simulink model "Canard"  (R2023b)
settings: Solver=ode4  StartTime=0.0  StopTime=30  FixedStep=Step_Size  RelTol=1e-3
values from neighbouring files (symbols this model uses):
  I_TENSOR = [ I_xx,  0.0, -I_xz ... (first row only)    [aircraft_dynamics.m]    (also in duomian.m; main.m; parameters.m)
  Init_Euler = [0 5 0]*d2r    [duomian.m]    (also in main.m; parameters.m)
  Init_Pos = [0 0 0]    [duomian.m]    (also in main.m; parameters.m)
  Init_Rate = [0 0 0]*d2r    [duomian.m]    (also in main.m; parameters.m)
  Init_Vel = [18.6923 0 1.6352]    [duomian.m]    (also in main.m; parameters.m)
  Mass = 18    [aircraft_dynamics.m]    (also in duomian.m; main.m; parameters.m)
  max_T = 97.02    [duomian.m]    (also in main.m; parameters.m)
  min_T = 0    [duomian.m]    (also in main.m; parameters.m)
undefined symbols (not defined in the file or in its folder): deg, e0_0, e1_0, e2_0, e3_0, Earth, rad, s, WGS84
libraries: aerolibconvert2 x5, shared6dof x4, aerolibasang x4, sharedtransform x3, slpidlib x1, shared6dofsys x1, sharedutil x1, aerolibtransform2 x1, aerolibatmos2 x1
settings Model: PauseTimes=0.01  Creator=11851  LastModifiedBy=11851
settings DataIOCC: ExternalInput=getinputstruct(op_trim5)  InitialState=getstatestruct(op_trim5)

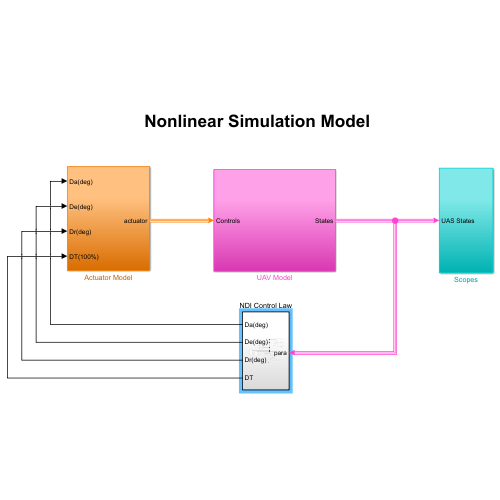
[thumbnail: Simulink's stored preview of the top-level diagram]
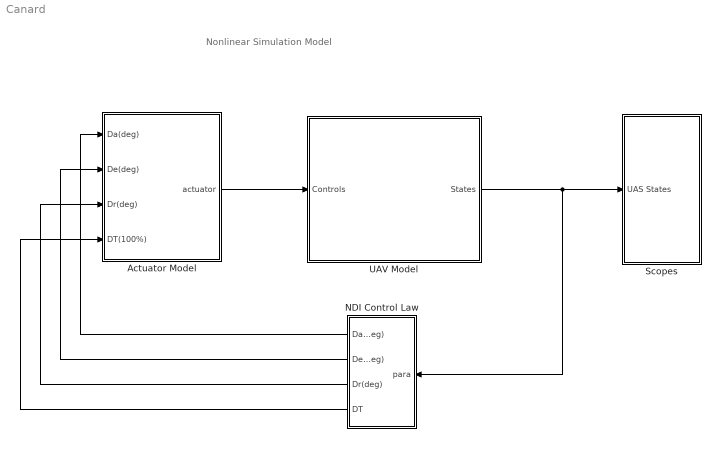
== system Canard ==
  note: Nonlinear Simulation Model
  Actuator Model : Subsystem
  NDI Control Law : Subsystem
  Scopes : Subsystem
  UAV Model : Subsystem
  wires:
  Actuator Model/1(actuator) -> UAV Model/1(Controls)
  UAV Model/1(States) -> NDI Control Law/1(para), Scopes/1(UAS States)
  NDI Control Law/1(Da(deg)) -> Actuator Model/1(Da(deg))
  NDI Control Law/2(De(deg)) -> Actuator Model/2(De(deg))
  NDI Control Law/3(Dr(deg)) -> Actuator Model/3(Dr(deg))
  NDI Control Law/4(DT) -> Actuator Model/4(DT(100%))

== system Canard/Actuator Model ==
  note: Actuator Models
  Da(deg) : Inport
  De(deg) : Inport  Port=2
  Dr(deg) : Inport  Port=3
  DT(100%) : Inport  Port=4
  Bus Creator : BusCreator  Inputs=2
  engine : Subsystem
  surface : Subsystem
  actuator : Outport
  wires:
  surface/1(control_surface(deg)) -> Bus Creator/1
  Bus Creator/1 -> actuator/1  "actuator"
  engine/1(throttle(100%)) -> Bus Creator/2
  Da(deg)/1 -> surface/1(Da(deg))
  De(deg)/1 -> surface/2(De(deg))
  DT(100%)/1 -> engine/1(DT(100%))
  Dr(deg)/1 -> surface/3(Dr(deg))

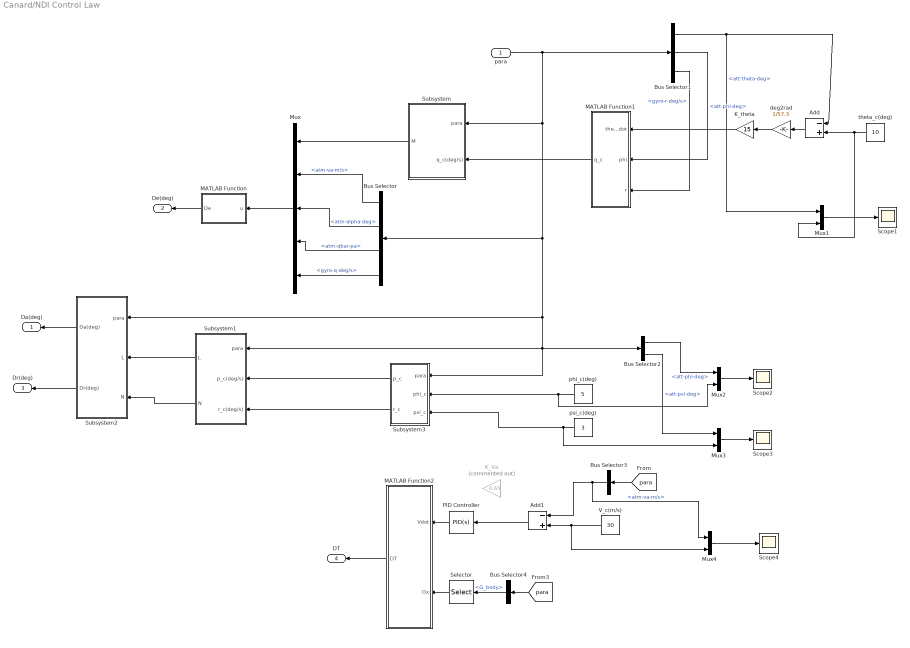
== system Canard/NDI Control Law ==
  para : Inport
  Add : Sum  Inputs=-+
  Add1 : Sum  Inputs=-+
  Bus Selector : BusSelector  OutputSignals=atm-va-m/s,atm-alpha-deg,atm-qbar-pa,gyro-q-deg/s
  Bus Selector1 : BusSelector  OutputSignals=att-theta-deg,att-phi-deg,gyro-r-deg/s
  Bus Selector2 : BusSelector  OutputSignals=att-phi-deg,att-psi-deg
  Bus Selector3 : BusSelector  OutputSignals=atm-va-m/s
  Bus Selector4 : BusSelector  OutputSignals=G_body
  K_Va : Gain  Commented=on  Gain=0.65
  K_theta : Gain  Gain=15
  MATLAB Function : MATLAB Function  TreatAsAtomicUnit=on
  MATLAB Function1 : MATLAB Function  TreatAsAtomicUnit=on
  MATLAB Function2 : MATLAB Function  TreatAsAtomicUnit=on
  Mux : Mux  Inputs=5
  Mux{1..4} (4 alike) : Mux  Inputs=2
  PID Controller : slpidlib/PID Controller  Controller=PID  Form=Parallel  TimeDomain=Continuous-time  UseExternalTs=off  SampleTime=-1  IntegratorMethod=Forward Euler  FilterMethod=Forward Euler  ControllerParametersSource=internal  P=0.75  I=0.05  UseKiTs=off  D=0  N=100  UseFilter=on  TunerSelectOption=Transfer Function Based (PID Tuner App)  InitialConditionSource=internal  InitialConditionForIntegrator=0  InitialConditionForFilter=0  DifferentiatorICPrevScaledInput=0  ExternalReset=none  TrackingMode=off  Kt=1  LimitOutput=off  SatLimitsSource=internal  UpperSaturationLimit=inf  LowerSaturationLimit=-inf  LinearizeAsGain=on  AntiWindupMode=none  Kb=1  LimitIntegrator=off  UpperIntegratorSaturationLimit=inf  LowerIntegratorSaturationLimit=-inf  POutMin=[]  POutMax=[]  IOutMin=[]  IOutMax=[]  DOutMin=[]  DOutMax=[]  NOutMin=[]  NOutMax=[]  SumOutMin=[]  SumOutMax=[]  SaturationOutMin=[]  SaturationOutMax=[]  PParamMin=[]  PParamMax=[]  IParamMin=[]  IParamMax=[]  DParamMin=[]  DParamMax=[]  NParamMin=[]  NParamMax=[]  KbParamMin=[]  KbParamMax=[]  KtParamMin=[]  KtParamMax=[]  KbOutMin=[]  KbOutMax=[]  KtOutMin=[]  KtOutMax=[]  IntegratorOutMin=[]  IntegratorOutMax=[]  FilterOutMin=[]  FilterOutMax=[]  SumI1OutMin=[]  SumI1OutMax=[]  SumI2OutMin=[]  SumI2OutMax=[]  SumI3OutMin=[]  SumI3OutMax=[]  SumI4OutMin=[]  SumI4OutMax=[]  SumDOutMin=[]  SumDOutMax=[]  DifferentiatorOutMin=[]  DifferentiatorOutMax=[]  FilterDiffOutCoefMin=[]  FilterDiffOutCoefMax=[]  ReciprocalOutMin=[]  ReciprocalOutMax=[]  SumDenOutMin=[]  SumDenOutMax=[]  SumNumOutMin=[]  SumNumOutMax=[]  DivideOutMin=[]  DivideOutMax=[]  UdiffTsProdOutMin=[]  UdiffTsProdOutMax=[]  NTsProdOutMin=[]  NTsProdOutMax=[]  UintegralTsProdOutMin=[]  UintegralTsProdOutMax=[]  UngainTsProdOutMin=[]  UngainTsProdOutMax=[]  ClampingZeroOutDataTypeStr=Inherit: Inherit via back propagation  ClampingZeroOutMin=[]  ClampingZeroOutMax=[]  FilterDenConstantOutDataTypeStr=Inherit: Inherit via back propagation  FilterDenConstantOutMin=[]  FilterDenConstantOutMax=[]  PCopyOutDataTypeStr=Inherit: Inherit via back propagation  PCopyOutMin=[]  PCopyOutMax=[]  NCopyOutDataTypeStr=Inherit: Inherit via back propagation  NCopyOutMin=[]  NCopyOutMax=[]  IntegratorContinuousStateAttributes=''  IntegratorStateMustResolveToSignalObject=off  IntegratorRTWStateStorageClass=Auto  FilterContinuousStateAttributes=''  FilterStateMustResolveToSignalObject=off  FilterRTWStateStorageClass=Auto  ParallelPVariant=InternalParameters  IdealPVariant=Disabled  IVariant=InternalParameters  DVariant=InternalParameters  IntegratorVariant=Continuous  SatVariant=Disabled  AWVariant=Passthrough  PCopyVariant=Disabled  TRVariant=Disabled  FdbkBlocksVariant=Forward  IdealPFdbkVariant=Disabled  SatFdbkVariant=Disabled  DerivativeFilterVariant=ContFilter  NVariant=InternalParameters  NCopyVariant=Disabled  FilterICVariant=InternalICsFilter  IntegratorICVariant=InternalICs  ExternalResetVariant=Disabled  TRSumVariant=Passthrough  SumFdbkVariant=Disabled  SumVariant=Sum_PID  TsampFilterVariant=InternalTs  TsampNgainVariant=Passthrough  TsampIntegralVariant=Disabled_SignalSpec  ExternalSaturationOutDataTypeStr=Inherit: Same as second input
  Scope{1..4} (4 alike) : Scope
  Selector : Selector  InputPortWidth=3  IndexOptions=Index vector (dialog)  Indices=1  OutputSizes=1
  Subsystem : Subsystem
  Subsystem1 : Subsystem
  Subsystem2 : Subsystem
  Subsystem3 : Subsystem
  V_c(m/s) : Constant  Value=30
  deg2rad : Gain  Gain=1/57.3
  phi_c(deg) : Constant  Value=5
  psi_c(deg) : Constant  Value=3
  theta_c(deg) : Constant  Value=10
  Da(deg) : Outport
  De(deg) : Outport  Port=2
  Dr(deg) : Outport  Port=3
  DT : Outport  Port=4
  wires:
  Subsystem1/2(N) -> Subsystem2/3(N)
  Mux4/1 -> Scope4/1
  Bus Selector2/1 -> Mux2/1  "<att-phi-deg>"
  Bus Selector1/1 -> Mux1/1, Add/1  "<att-theta-deg>"
  deg2rad/1 -> K_theta/1
  [para] -> Bus Selector3/1
  Bus Selector3/1 -> Mux4/1, Add1/1  "<atm-va-m/s>"
  para/1 -> Subsystem3/1(para), Bus Selector2/1, Subsystem1/1(para), Subsystem2/1(para), Bus Selector/1, Subsystem/1(para), Bus Selector1/1
  Bus Selector2/2 -> Mux3/1  "<att-psi-deg>"
  Subsystem1/1(L) -> Subsystem2/2(L)
  Add/1 -> deg2rad/1
  Subsystem/1(M) -> Mux/1
  theta_c(deg)/1 -> Mux1/2, Add/2
  Bus Selector1/3 -> MATLAB Function1/3(r)  "<gyro-r-deg/s>"
  Subsystem3/2(r_c) -> Subsystem1/3(r_c(deg/s))
  Mux2/1 -> Scope2/1
  Mux1/1 -> Scope1/1
  K_theta/1 -> MATLAB Function1/1(thetac_dot)
  MATLAB Function1/1(q_c) -> Subsystem/2(q_c(deg/s))
  [para] -> Bus Selector4/1
  psi_c(deg)/1 -> Mux3/2, Subsystem3/3(psi_c)
  Bus Selector/4 -> Mux/5  "<gyro-q-deg/s>"
  Mux/1 -> MATLAB Function/1(u)
  Subsystem3/1(p_c) -> Subsystem1/2(p_c(deg/s))
  Bus Selector/2 -> Mux/3  "<atm-alpha-deg>"
  Mux3/1 -> Scope3/1
  phi_c(deg)/1 -> Mux2/2, Subsystem3/2(phi_c)
  Bus Selector4/1 -> Selector/1  "<G_body>"
  Bus Selector/3 -> Mux/4  "<atm-qbar-pa>"
  Bus Selector1/2 -> MATLAB Function1/2(phi)  "<att-phi-deg>"
  Bus Selector/1 -> Mux/2  "<atm-va-m/s>"
  V_c(m/s)/1 -> Mux4/2, Add1/2
  Selector/1 -> MATLAB Function2/2(Gx)
  MATLAB Function2/1(DT) -> DT/1
  Subsystem2/2(Dr(deg)) -> Dr(deg)/1
  MATLAB Function/1(De) -> De(deg)/1
  Subsystem2/1(Da(deg)) -> Da(deg)/1
  Add1/1 -> PID Controller/1
  PID Controller/1 -> MATLAB Function2/1(Vdot)

== system Canard/Scopes ==
  UAS States : Inport
  Bus Selector : BusSelector  OutputSignals=att-phi-deg,att-theta-deg,att-psi-deg,gyro-p-deg/s,gyro-q-deg/s,gyro-r-deg/s,atm-va-m/s,atm-alpha-deg,atm-beta-deg
  Euler : Scope  NumInputPorts=3
  Vabs : Scope
  alpha_beta : Scope  NumInputPorts=2
  pqr : Scope  NumInputPorts=3
  wires:
  UAS States/1 -> Bus Selector/1
  Bus Selector/1 -> Euler/1  "<att-phi-deg>"
  Bus Selector/2 -> Euler/2  "<att-theta-deg>"
  Bus Selector/3 -> Euler/3  "<att-psi-deg>"
  Bus Selector/4 -> pqr/1  "<gyro-p-deg/s>"
  Bus Selector/5 -> pqr/2  "<gyro-q-deg/s>"
  Bus Selector/6 -> pqr/3  "<gyro-r-deg/s>"
  Bus Selector/7 -> Vabs/1  "<atm-va-m/s>"
  Bus Selector/8 -> alpha_beta/1  "<atm-alpha-deg>"
  Bus Selector/9 -> alpha_beta/2  "<atm-beta-deg>"

== system Canard/UAV Model ==
  note: Dynamics Model
  Controls : Inport
  Aerodynamics : Subsystem
  Bus Creator : BusCreator  Inputs=2
  Equations of Motion : Subsystem
  Propulsive Force & Moment : Subsystem
  Total Force & Moment : Subsystem
  environment : Subsystem
  gravitation : Subsystem
  States : Outport
  tag scope: para=global
  wires:
  Aerodynamics/1(fxyz) -> Total Force & Moment/1(F_aero)
  Aerodynamics/2(mxyz) -> Total Force & Moment/2(M_aero)
  Controls/1 -> Propulsive Force & Moment/1(Controls), Bus Creator/1
  Propulsive Force & Moment/1(F_prop) -> Total Force & Moment/3(F_prop)
  Propulsive Force & Moment/2(M_prop) -> Total Force & Moment/4(M_prop)
  Total Force & Moment/1(F_cg) -> Equations of Motion/1(Force)
  Total Force & Moment/2(M_cg) -> Equations of Motion/2(Moment)
  Equations of Motion/1(para) -> States/1, Bus Creator/2, gravitation/1(state), [para]
  gravitation/1(gravity) -> Total Force & Moment/5(gravity)
  gravitation/2(moment) -> Total Force & Moment/6(M_grav)
  Bus Creator/1 -> Aerodynamics/1(state)

== system Canard/Actuator Model/engine ==
  note: 发动机油门开合度
  DT(100%) : Inport
  Gain : Gain  Gain=10
  Integrator : Integrator  InitialConditionSource=external
  Saturation1 : Saturate  UpperLimit=300  LowerLimit=-300
  Saturation2 : Saturate  UpperLimit=1  LowerLimit=0
  Sum : Sum  Inputs=|+-
  throttle(100%) : Outport
  wires:
  Integrator/1 -> Saturation2/1
  Saturation1/1 -> Integrator/1
  Gain/1 -> Saturation1/1
  Sum/1 -> Gain/1
  DT(100%)/1 -> Sum/1, Integrator/2
  Saturation2/1 -> throttle(100%)/1, Sum/2  "throttle"

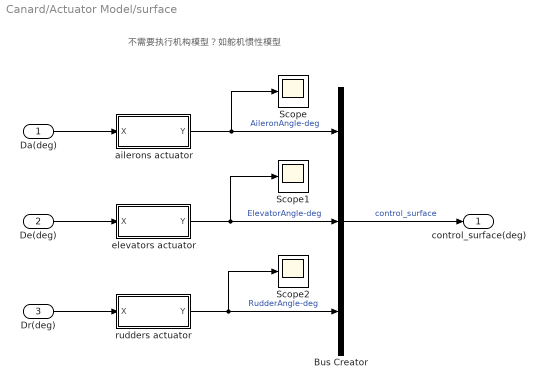
== system Canard/Actuator Model/surface ==
  note: 不需要执行机构模型？如舵机惯性模型
  Da(deg) : Inport
  De(deg) : Inport  Port=2
  Dr(deg) : Inport  Port=3
  Bus Creator : BusCreator  Inputs=3
  Scope : Scope
  Scope1 : Scope
  Scope2 : Scope
  ailerons actuator : Subsystem
  elevators actuator : Subsystem
  rudders actuator : Subsystem
  control_surface(deg) : Outport
  wires:
  Bus Creator/1 -> control_surface(deg)/1  "control_surface"
  ailerons actuator/1(Y) -> Scope/1, Bus Creator/1  "AileronAngle-deg"
  elevators actuator/1(Y) -> Scope1/1, Bus Creator/2  "ElevatorAngle-deg"
  rudders actuator/1(Y) -> Scope2/1, Bus Creator/3  "RudderAngle-deg"
  Da(deg)/1 -> ailerons actuator/1(X)
  De(deg)/1 -> elevators actuator/1(X)
  Dr(deg)/1 -> rudders actuator/1(X)

== system Canard/NDI Control Law/Subsystem ==
  para : Inport
  q_c(deg/s) : Inport  Port=2
  Add : Sum  Inputs=-+
  Bus Selector : BusSelector  OutputSignals=gyro-p-deg/s,gyro-q-deg/s,gyro-r-deg/s
  K_q : Gain  Gain=5
  MATLAB Function : MATLAB Function  TreatAsAtomicUnit=on
  deg2rad : Gain  Gain=1/57.3
  deg2rad1 : Gain  Gain=1/57.3
  deg2rad2 : Gain  Gain=1/57.3
  M : Outport
  wires:
  para/1 -> Bus Selector/1
  Bus Selector/2 -> Add/1  "<gyro-q-deg/s>"
  q_c(deg/s)/1 -> Add/2
  deg2rad/1 -> K_q/1
  Add/1 -> deg2rad/1
  K_q/1 -> MATLAB Function/3(q_dot)
  Bus Selector/1 -> deg2rad2/1  "<gyro-p-deg/s>"
  Bus Selector/3 -> deg2rad1/1  "<gyro-r-deg/s>"
  MATLAB Function/1(M) -> M/1
  deg2rad2/1 -> MATLAB Function/1(p)
  deg2rad1/1 -> MATLAB Function/2(r)

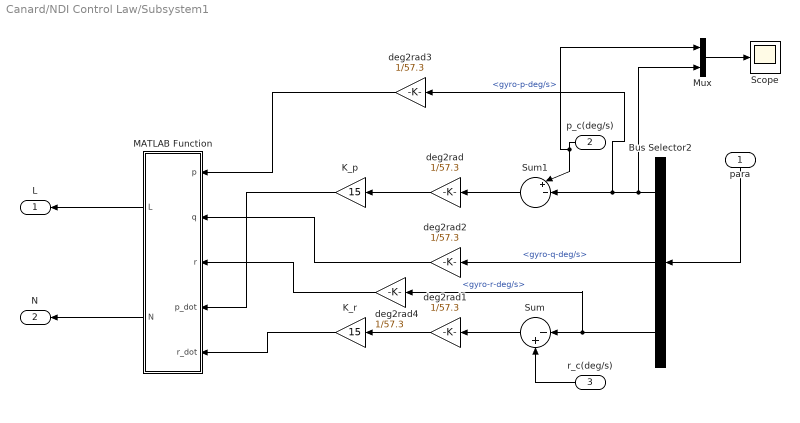
== system Canard/NDI Control Law/Subsystem1 ==
  para : Inport
  p_c(deg/s) : Inport  Port=2
  r_c(deg/s) : Inport  Port=3
  Bus Selector2 : BusSelector  OutputSignals=gyro-p-deg/s,gyro-q-deg/s,gyro-r-deg/s
  K_p : Gain  Gain=15
  K_r : Gain  Gain=15
  MATLAB Function : MATLAB Function  TreatAsAtomicUnit=on
  Mux : Mux  Inputs=2
  Scope : Scope
  Sum : Sum  Inputs=|-+
  Sum1 : Sum  Inputs=|+-||
  deg2rad{,1..4} (5 alike) : Gain  Gain=1/57.3
  L : Outport
  N : Outport  Port=2
  wires:
  Bus Selector2/2 -> deg2rad2/1  "<gyro-q-deg/s>"
  r_c(deg/s)/1 -> Sum/2
  para/1 -> Bus Selector2/1
  deg2rad1/1 -> K_r/1
  deg2rad/1 -> K_p/1
  Bus Selector2/1 -> Mux/2, deg2rad3/1, Sum1/2  "<gyro-p-deg/s>"
  Bus Selector2/3 -> deg2rad4/1, Sum/1  "<gyro-r-deg/s>"
  Sum1/1 -> deg2rad/1
  Sum/1 -> deg2rad1/1
  p_c(deg/s)/1 -> Sum1/1, Mux/1
  deg2rad3/1 -> MATLAB Function/1(p)
  deg2rad2/1 -> MATLAB Function/2(q)
  deg2rad4/1 -> MATLAB Function/3(r)
  K_p/1 -> MATLAB Function/4(p_dot)
  K_r/1 -> MATLAB Function/5(r_dot)
  MATLAB Function/1(L) -> L/1
  MATLAB Function/2(N) -> N/1
  Mux/1 -> Scope/1

== system Canard/NDI Control Law/Subsystem2 ==
  para : Inport
  L : Inport  Port=2
  N : Inport  Port=3
  Bus Selector2 : BusSelector  OutputSignals=atm-qbar-pa,atm-alpha-deg,atm-beta-deg,atm-va-m/s,gyro-p-deg/s,gyro-r-deg/s
  MATLAB Function : MATLAB Function  TreatAsAtomicUnit=on
  Da(deg) : Outport
  Dr(deg) : Outport  Port=2
  wires:
  para/1 -> Bus Selector2/1
  Bus Selector2/1 -> MATLAB Function/1(qbar)  "<atm-qbar-pa>"
  Bus Selector2/2 -> MATLAB Function/2(alpha)  "<atm-alpha-deg>"
  Bus Selector2/4 -> MATLAB Function/4(va)  "<atm-va-m/s>"
  Bus Selector2/3 -> MATLAB Function/3(beta)  "<atm-beta-deg>"
  Bus Selector2/6 -> MATLAB Function/6(r)  "<gyro-r-deg/s>"
  Bus Selector2/5 -> MATLAB Function/5(p)  "<gyro-p-deg/s>"
  L/1 -> MATLAB Function/7(L)
  N/1 -> MATLAB Function/8(N)
  MATLAB Function/2(Dr) -> Dr(deg)/1
  MATLAB Function/1(Da) -> Da(deg)/1

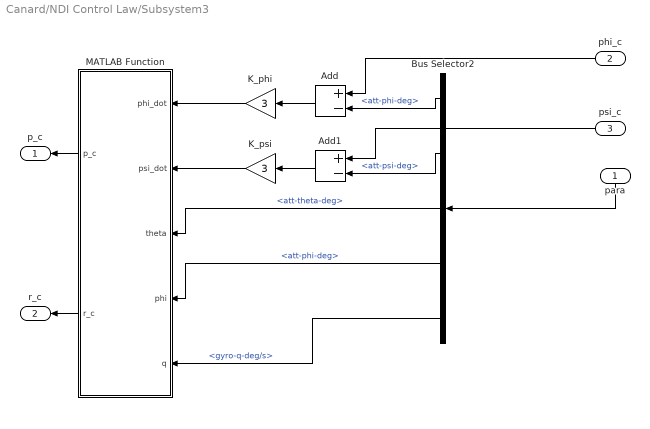
== system Canard/NDI Control Law/Subsystem3 ==
  para : Inport
  phi_c : Inport  Port=2
  psi_c : Inport  Port=3
  Add : Sum  Inputs=+-
  Add1 : Sum  Inputs=+-
  Bus Selector2 : BusSelector  OutputSignals=att-phi-deg,att-psi-deg,att-theta-deg,att-phi-deg,gyro-q-deg/s
  K_phi : Gain  Gain=3
  K_psi : Gain  Gain=3
  MATLAB Function : MATLAB Function  TreatAsAtomicUnit=on
  p_c : Outport
  r_c : Outport  Port=2
  wires:
  Bus Selector2/5 -> MATLAB Function/5(q)  "<gyro-q-deg/s>"
  para/1 -> Bus Selector2/1
  Bus Selector2/1 -> Add/2  "<att-phi-deg>"
  Bus Selector2/2 -> Add1/2  "<att-psi-deg>"
  Bus Selector2/3 -> MATLAB Function/3(theta)  "<att-theta-deg>"
  phi_c/1 -> Add/1
  Add/1 -> K_phi/1
  psi_c/1 -> Add1/1
  Add1/1 -> K_psi/1
  Bus Selector2/4 -> MATLAB Function/4(phi)  "<att-phi-deg>"
  MATLAB Function/1(p_c) -> p_c/1
  MATLAB Function/2(r_c) -> r_c/1
  K_phi/1 -> MATLAB Function/1(phi_dot)
  K_psi/1 -> MATLAB Function/2(psi_dot)

== system Canard/UAV Model/Aerodynamics ==
  note: Aerodynamics Module
  state : Inport
  Bus Selector : BusSelector  OutputSignals=actuator.control_surface.AileronAngle-deg,actuator.control_surface.ElevatorAngle-deg,actuator.control_surface.RudderAngle-deg,para.atm-alpha-deg,para.atm-beta-deg,para.gyro-p-deg/s,para.gyro-q-deg/s,para.gyro-r-deg/s,para.atm-va-m/s,para.atm-qbar-pa
  Demux : Demux  Outputs=6
  Mux : Mux  Inputs=10
  Mux1 : Mux  Inputs=3
  Mux2 : Mux  Inputs=3
  S-Function : S-Function  FunctionName=Canard_aero  SFunctionDeploymentMode=off  EnableBusSupport=off
  fxyz : Outport
  mxyz : Outport  Port=2
  wires:
  Bus Selector/9 -> Mux/9  "<atm-va-m/s>"
  Bus Selector/10 -> Mux/10  "<atm-qbar-pa>"
  Bus Selector/1 -> Mux/1  "<AileronAngle-deg>"
  Demux/2 -> Mux1/2
  Mux2/1 -> mxyz/1
  Demux/3 -> Mux1/3
  Demux/6 -> Mux2/3
  Bus Selector/5 -> Mux/5  "<atm-beta-deg>"
  Mux1/1 -> fxyz/1
  Demux/4 -> Mux2/1
  Mux/1 -> S-Function/1
  S-Function/1 -> Demux/1
  state/1 -> Bus Selector/1
  Bus Selector/2 -> Mux/2  "<ElevatorAngle-deg>"
  Demux/5 -> Mux2/2
  Bus Selector/7 -> Mux/7  "<gyro-q-deg/s>"
  Bus Selector/4 -> Mux/4  "<atm-alpha-deg>"
  Demux/1 -> Mux1/1
  Bus Selector/6 -> Mux/6  "<gyro-p-deg/s>"
  Bus Selector/3 -> Mux/3  "<RudderAngle-deg>"
  Bus Selector/8 -> Mux/8  "<gyro-r-deg/s>"

== system Canard/UAV Model/Equations of Motion ==
  note: 6DOF Motion of Equations
  Force : Inport  PortDimensions=3
  Moment : Inport  Port=2  PortDimensions=3
  Subsystem : Subsystem
  parameter : Subsystem
  para : Outport
  wires:
  Moment/1 -> Subsystem/2(Moments)
  Force/1 -> Subsystem/1(Forces)
  Subsystem/1(Ve) -> parameter/1(Ve)
  Subsystem/2(Xe) -> parameter/2(Xe)
  Subsystem/3(Euler) -> parameter/3(Euler)
  Subsystem/4(DCM) -> parameter/4(Rbe)
  Subsystem/5(Vb) -> parameter/5(Vb)
  Subsystem/6(p,q,r) -> parameter/6(ω)
  Subsystem/7(pdot,qdot,rdot) -> parameter/7(dω)
  Subsystem/8(Ab) -> parameter/8(Ab)
  parameter/1(para) -> para/1

== system Canard/UAV Model/Propulsive Force & Moment ==
  note: Propulsive Force and Moment
  Controls : Inport
  Bus Selector : BusSelector  OutputSignals=throttle
  Constant : Constant  Value=0
  Mux : Mux  Inputs=3
  Mux1 : Mux  Inputs=3
  Saturation : Saturate  UpperLimit=max_T  LowerLimit=min_T
  max_T : Gain  Gain=max_T
  F_prop : Outport
  M_prop : Outport  Port=2
  wires:
  Mux1/1 -> M_prop/1
  Constant/1 -> Mux1/3, Mux1/2, Mux1/1, Mux/3, Mux/2
  Controls/1 -> Bus Selector/1
  Mux/1 -> F_prop/1
  Saturation/1 -> Mux/1
  max_T/1 -> Saturation/1
  Bus Selector/1 -> max_T/1  "<throttle>"

== system Canard/UAV Model/Total Force & Moment ==
  note: Total Force and Moment
  F_aero : Inport  PortDimensions=3
  M_aero : Inport  Port=2  PortDimensions=3
  F_prop : Inport  Port=3  PortDimensions=3
  M_prop : Inport  Port=4  PortDimensions=3
  gravity : Inport  Port=5  PortDimensions=3
  M_grav : Inport  Port=6  PortDimensions=3
  Total Force : Sum  Inputs=+++  InputSameDT=on  SaturateOnIntegerOverflow=on  OutDataTypeStr=Inherit: Same as first input
  Total Moment : Sum  Inputs=+++  InputSameDT=on  SaturateOnIntegerOverflow=on  OutDataTypeStr=Inherit: Same as first input
  F_cg : Outport
  M_cg : Outport  Port=2
  wires:
  Total Force/1 -> F_cg/1
  F_aero/1 -> Total Force/1
  F_prop/1 -> Total Force/2
  M_prop/1 -> Total Moment/2
  Total Moment/1 -> M_cg/1
  M_aero/1 -> Total Moment/1
  gravity/1 -> Total Force/3
  M_grav/1 -> Total Moment/3

== system Canard/UAV Model/environment ==
  note: 物理环境模块，用于模拟飞机所处的环境，包括
      |
      | （1）标准大气模型
      | （2）风场运动模型，比如风切变等
      | （3）重力场模型
      | （4）磁力场模型
  Bus Creator1 : BusCreator  Inputs=4
  atmosphere : Subsystem
  gravity : Subsystem
  magnetic : Subsystem
  windshear : Subsystem
  tag scope: environment=global
  wires:
  Bus Creator1/1 -> [environment]  "Environment"
  atmosphere/1(atmo) -> Bus Creator1/1  "atmo"
  windshear/1(wind) -> Bus Creator1/2  "wind"
  gravity/1(g) -> Bus Creator1/3  "g"
  magnetic/1(mag) -> Bus Creator1/4  "mag"

== system Canard/UAV Model/gravitation ==
  state : Inport
  Bus Selector : BusSelector  OutputSignals=att-theta-deg,att-phi-deg
  Constant : Constant  Value=Mass
  Constant1 : Constant  Value=9.81
  MATLAB Function : MATLAB Function  TreatAsAtomicUnit=on
  Mux : Mux  Inputs=3
  Mux1 : Mux  Inputs=3
  Product : Product
  zero1 : Constant  Value=[0 0 0]
  gravity : Outport
  moment : Outport  Port=2
  wires:
  zero1/1 -> moment/1
  state/1 -> Bus Selector/1
  Bus Selector/1 -> Mux/2  "<att-theta-deg>"
  Bus Selector/2 -> Mux/3  "<att-phi-deg>"
  Constant/1 -> Product/1
  Product/1 -> Mux/1
  Mux/1 -> MATLAB Function/1(u)
  MATLAB Function/1(Gx) -> Mux1/1
  MATLAB Function/2(Gy) -> Mux1/2
  MATLAB Function/3(Gz) -> Mux1/3
  Mux1/1 -> gravity/1
  Constant1/1 -> Product/2

== system Canard/Actuator Model/surface/ailerons actuator ==
  X : Inport
  Gain : Gain  Gain=100
  Integrator : Integrator  InitialConditionSource=external
  Saturation1 : Saturate  UpperLimit=300  LowerLimit=-300
  Saturation2 : Saturate  UpperLimit=20  LowerLimit=-20
  Sum : Sum  Inputs=|+-
  Y : Outport
  wires:
  Integrator/1 -> Saturation2/1
  Saturation1/1 -> Integrator/1
  Gain/1 -> Saturation1/1
  Sum/1 -> Gain/1
  Saturation2/1 -> Y/1, Sum/2
  X/1 -> Sum/1, Integrator/2

== system Canard/Actuator Model/surface/elevators actuator ==
  X : Inport
  Gain : Gain  Gain=100
  Integrator : Integrator  InitialConditionSource=external  InitialCondition=0.811
  Saturation1 : Saturate  UpperLimit=300  LowerLimit=-300
  Saturation2 : Saturate  UpperLimit=20  LowerLimit=-20
  Scope : Scope
  Sum : Sum  Inputs=|+-
  Y : Outport
  wires:
  Integrator/1 -> Saturation2/1
  Saturation1/1 -> Integrator/1
  Gain/1 -> Saturation1/1
  Sum/1 -> Gain/1
  Saturation2/1 -> Scope/1, Y/1, Sum/2
  X/1 -> Integrator/2, Sum/1

== system Canard/Actuator Model/surface/rudders actuator ==
  X : Inport
  Gain : Gain  Gain=100
  Integrator : Integrator  InitialConditionSource=external
  Saturation1 : Saturate  UpperLimit=300  LowerLimit=-300
  Saturation2 : Saturate  UpperLimit=20  LowerLimit=-20
  Sum : Sum  Inputs=|+-
  Y : Outport
  wires:
  Integrator/1 -> Saturation2/1
  Saturation1/1 -> Integrator/1
  Gain/1 -> Saturation1/1
  Sum/1 -> Gain/1
  Saturation2/1 -> Y/1, Sum/2
  X/1 -> Sum/1, Integrator/2

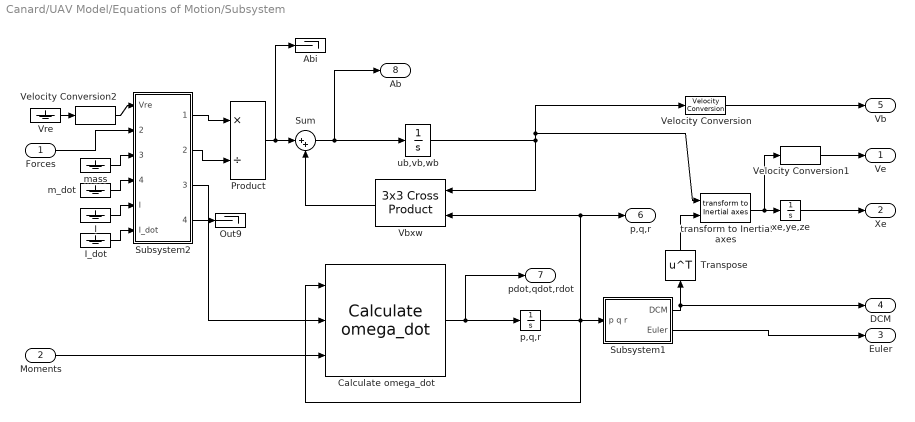
== system Canard/UAV Model/Equations of Motion/Subsystem ==
  Forces : Inport  OutDataTypeStr=double  Unit=N  PortDimensions=3
  Moments : Inport  Port=2  OutDataTypeStr=double  Unit=N*m  PortDimensions=3
  Abi : Terminator
  Calculate omega_dot : shared6dofsys/Calculate omega_dot  aMode=aMode
  I : Ground
  I_dot : Ground
  Out9 : Terminator
  Product : Product  Inputs=*/  SaturateOnIntegerOverflow=on  OutDataTypeStr=Inherit: Same as first input
  Subsystem1 : Subsystem
  Subsystem2 : Subsystem
  Sum : Sum  Inputs=|++  SaturateOnIntegerOverflow=on
  Transpose : Math  Operator=transpose  SignedPower=on
  Vbxw : sharedutil/3x3 Cross Product  aMode=aMode
  Velocity Conversion : shared6dof/6DOF (Euler Angles)/Velocity Conversion  SystemSampleTime=-1  VariantActivationTime=update diagram  AllowFlexibleInterface=on  Latency=0  AutoFrameSizeCalculation=off
  Velocity Conversion1 : shared6dof/6DOF (Euler Angles)/Velocity Conversion1  SystemSampleTime=-1  VariantActivationTime=update diagram  AllowFlexibleInterface=on  Latency=0  AutoFrameSizeCalculation=off
  Velocity Conversion2 : shared6dof/6DOF (Euler Angles)/Velocity Conversion2  SystemSampleTime=-1  VariantActivationTime=update diagram  AllowFlexibleInterface=on  Latency=0  AutoFrameSizeCalculation=off
  Vre : Ground
  m_dot : Ground
  mass : Ground
  "p,q,r " : Integrator  InitialCondition=Init_Rate
  "transform to Inertial axes " : shared6dof/6DOF (Euler Angles)/transform to Inertial axes   SystemSampleTime=-1  VariantActivationTime=update diagram  AllowFlexibleInterface=on  Latency=0  AutoFrameSizeCalculation=off
  ub,vb,wb : Integrator  InitialCondition=Init_Vel
  xe,ye,ze : Integrator  InitialCondition=Init_Pos
  Ve : Outport  OutDataTypeStr=double  Unit=m/s  VectorParamsAs1DForOutWhenUnconnected=off
  Xe : Outport  Port=2  OutDataTypeStr=double  Unit=m  VectorParamsAs1DForOutWhenUnconnected=off
  Euler : Outport  Port=3  OutDataTypeStr=double  Unit=rad  VectorParamsAs1DForOutWhenUnconnected=off
  DCM : Outport  Port=4  OutDataTypeStr=double  Unit=1  VectorParamsAs1DForOutWhenUnconnected=off
  Vb : Outport  Port=5  OutDataTypeStr=double  Unit=m/s  VectorParamsAs1DForOutWhenUnconnected=off
  p,q,r : Outport  Port=6  OutDataTypeStr=double  Unit=rad/s  VectorParamsAs1DForOutWhenUnconnected=off
  pdot,qdot,rdot : Outport  Port=7  OutDataTypeStr=double  Unit=rad/s^2  VectorParamsAs1DForOutWhenUnconnected=off
  Ab : Outport  Port=8  OutDataTypeStr=double  Unit=m/s^2  VectorParamsAs1DForOutWhenUnconnected=off
  wires:
  Transpose/1 -> "transform to Inertial axes "/2
  ub,vb,wb/1 -> Vbxw/1, Velocity Conversion/1, "transform to Inertial axes "/1
  m_dot/1 -> Subsystem2/4(m_dot)
  Calculate omega_dot/1 -> pdot,qdot,rdot/1, "p,q,r "/1
  I_dot/1 -> Subsystem2/6(I_dot)
  Forces/1 -> Subsystem2/2(forces)
  Product/1 -> Sum/1, Abi/1
  "p,q,r "/1 -> Calculate omega_dot/1, Subsystem1/1(p q r), p,q,r/1, Vbxw/2
  Vbxw/1 -> Sum/2
  Subsystem2/1("forces ") -> Product/1
  Sum/1 -> Ab/1, ub,vb,wb/1
  Moments/1 -> Calculate omega_dot/3
  Velocity Conversion/1 -> Vb/1
  Subsystem1/1(DCM) -> DCM/1, Transpose/1
  Subsystem1/2(Euler) -> Euler/1
  Velocity Conversion1/1 -> Ve/1
  mass/1 -> Subsystem2/3("mass ")
  Velocity Conversion2/1 -> Subsystem2/1(Vre)
  Vre/1 -> Velocity Conversion2/1
  "transform to Inertial axes "/1 -> xe,ye,ze/1, Velocity Conversion1/1
  xe,ye,ze/1 -> Xe/1
  I/1 -> Subsystem2/5(I)
  Subsystem2/4(Out9) -> Out9/1
  Subsystem2/3("inertia, 0") -> Calculate omega_dot/2
  Subsystem2/2(mass) -> Product/2

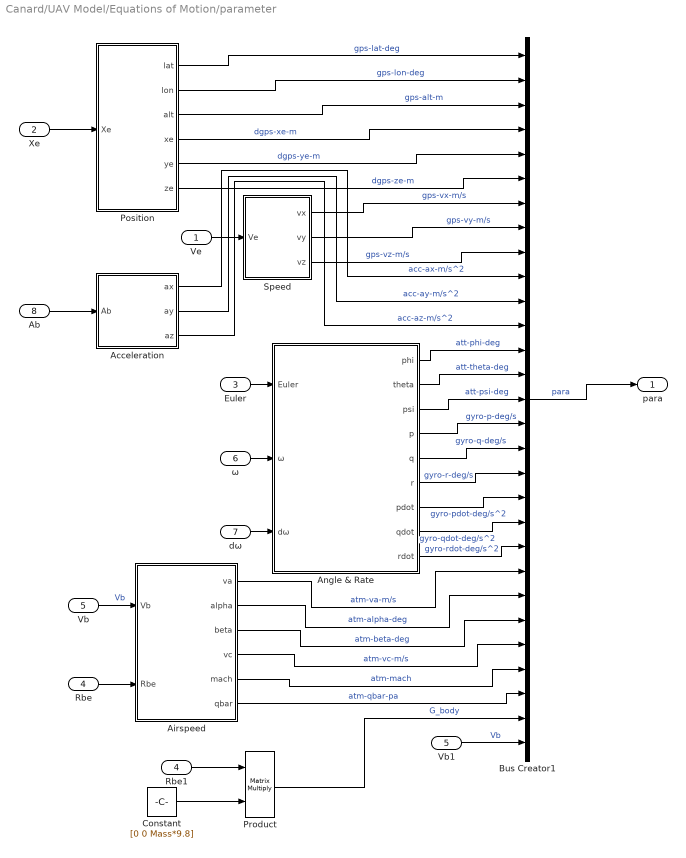
== system Canard/UAV Model/Equations of Motion/parameter ==
  Ve : Inport
  Xe : Inport  Port=2
  Euler : Inport  Port=3
  Rbe : Inport  Port=4
  Vb : Inport  Port=5
  ω : Inport  Port=6
  dω : Inport  Port=7
  Ab : Inport  Port=8
  Acceleration : Subsystem
  Airspeed : Subsystem
  Angle & Rate : Subsystem
  Bus Creator1 : BusCreator  Inputs=29
  Constant : Constant  Value=[0 0 Mass*9.8]
  "Position " : Subsystem
  Product : Product  Multiplication=Matrix(*)
  Rbe1 : InportShadow  Port=4
  Speed : Subsystem
  Vb1 : InportShadow  Port=5
  para : Outport
  wires:
  Bus Creator1/1 -> para/1  "para"
  Euler/1 -> Angle & Rate/1(Euler)
  ω/1 -> Angle & Rate/2(ω)
  dω/1 -> Angle & Rate/3(dω)
  Vb/1 -> Airspeed/1(Vb)  "Vb"
  Rbe/1 -> Airspeed/2(Rbe)
  Ab/1 -> Acceleration/1(Ab)
  Ve/1 -> Speed/1(Ve)
  Xe/1 -> "Position "/1(Xe)
  "Position "/1(lat) -> Bus Creator1/1  "gps-lat-deg"
  "Position "/2(lon) -> Bus Creator1/2  "gps-lon-deg"
  "Position "/3(alt) -> Bus Creator1/3  "gps-alt-m"
  "Position "/4(xe) -> Bus Creator1/4  "dgps-xe-m"
  "Position "/5(ye) -> Bus Creator1/5  "dgps-ye-m"
  "Position "/6(ze) -> Bus Creator1/6  "dgps-ze-m"
  Speed/1(vx) -> Bus Creator1/7  "gps-vx-m/s"
  Speed/2(vy) -> Bus Creator1/8  "gps-vy-m/s"
  Speed/3(vz) -> Bus Creator1/9  "gps-vz-m/s"
  Acceleration/1(ax) -> Bus Creator1/10  "acc-ax-m/s^2"
  Acceleration/2(ay) -> Bus Creator1/11  "acc-ay-m/s^2"
  Acceleration/3(az) -> Bus Creator1/12  "acc-az-m/s^2"
  Angle & Rate/1(phi) -> Bus Creator1/13  "att-phi-deg"
  Angle & Rate/2(theta) -> Bus Creator1/14  "att-theta-deg"
  Angle & Rate/3(psi) -> Bus Creator1/15  "att-psi-deg"
  Angle & Rate/4(p) -> Bus Creator1/16  "gyro-p-deg/s"
  Angle & Rate/5(q) -> Bus Creator1/17  "gyro-q-deg/s"
  Angle & Rate/6(r) -> Bus Creator1/18  "gyro-r-deg/s"
  Angle & Rate/7(pdot) -> Bus Creator1/19  "gyro-pdot-deg/s^2"
  Angle & Rate/8(qdot) -> Bus Creator1/20  "gyro-qdot-deg/s^2"
  Angle & Rate/9(rdot) -> Bus Creator1/21  "gyro-rdot-deg/s^2"
  Airspeed/1(va) -> Bus Creator1/22  "atm-va-m/s"
  Airspeed/2(alpha) -> Bus Creator1/23  "atm-alpha-deg"
  Airspeed/3(beta) -> Bus Creator1/24  "atm-beta-deg"
  Airspeed/4(vc) -> Bus Creator1/25  "atm-vc-m/s"
  Airspeed/5(mach) -> Bus Creator1/26  "atm-mach"
  Airspeed/6(qbar) -> Bus Creator1/27  "atm-qbar-pa"
  Rbe1/1 -> Product/1
  Constant/1 -> Product/2
  Product/1 -> Bus Creator1/28  "G_body"
  Vb1/1 -> Bus Creator1/29  "Vb"

== system Canard/UAV Model/environment/atmosphere ==
  Bus Creator : BusCreator  Inputs=4
  COESA Atmosphere Model : aerolibatmos2/COESA Atmosphere Model  units=Metric (MKS)  spec=1976 COESA-extended U.S. Standard Atmosphere  model=Profile  profile_var=High temperature  profile_percent=1%  profile_alt=5 km (16404 ft)  envelope_var=High temperature  envelope_percent=1%  action=Warning
  atmo : Outport
  wires:
  Bus Creator/1 -> atmo/1
  COESA Atmosphere Model/3 -> Bus Creator/3  "AirPress-Pa"
  COESA Atmosphere Model/1 -> Bus Creator/1  "temp-K"
  COESA Atmosphere Model/2 -> Bus Creator/2  "SoundSpeed"
  COESA Atmosphere Model/4 -> Bus Creator/4  "AirDens-kg/m^3"
  [height] -> COESA Atmosphere Model/1

== system Canard/UAV Model/environment/gravity ==
  g-m/s^2 : Constant  Value=9.8
  g : Outport
  tag scope: g=global
  wires:
  g-m/s^2/1 -> [g], g/1

== system Canard/UAV Model/environment/magnetic ==
  Constant : Constant  Value=[1 1 1]
  mag : Outport
  wires:
  Constant/1 -> mag/1

== system Canard/UAV Model/environment/windshear ==
  Constant : Constant  Value=[0 0 0]
  wind : Outport
  wires:
  Constant/1 -> wind/1

== system Canard/UAV Model/Equations of Motion/Subsystem/Subsystem1 ==
  p q r : Inport  OutDataTypeStr=double
  Initial Euler Angles : Constant  Value=Init_Euler
  Quaternions to Direction Cosine Matrix : sharedtransform/Quaternions to  Direction Cosine Matrix  aMode=aMode
  Quaternions to Rotation Angles : sharedtransform/Quaternions to Rotation Angles  rotationOrder=ZYX  aMode=aMode
  Rotation Angles to Quaternions : sharedtransform/Rotation Angles to Quaternions  rotationOrder=ZYX  aMode=aMode
  Selector : Selector  InputPortWidth=3  IndexOptions=Index vector (dialog)  Indices=[3 2 1]  OutputSizes=1
  Selector1 : Selector  InputPortWidth=3  IndexOptions=Index vector (dialog)  Indices=[3 2 1]  OutputSizes=1
  Subsystem3 : Subsystem
  q0 q1 q2 q3 : Integrator  InitialConditionSource=external  InitialCondition=[e0_0 e1_0 e2_0 e3_0]
  DCM : Outport  OutDataTypeStr=double  VectorParamsAs1DForOutWhenUnconnected=off
  Euler : Outport  Port=2  OutDataTypeStr=double  VectorParamsAs1DForOutWhenUnconnected=off
  wires:
  Selector1/1 -> Rotation Angles to Quaternions/1
  Rotation Angles to Quaternions/1 -> q0 q1 q2 q3/2
  Subsystem3/1(qdot) -> q0 q1 q2 q3/1
  q0 q1 q2 q3/1 -> Subsystem3/2(q0 q1 q2 q3), Quaternions to Rotation Angles/1, Quaternions to Direction Cosine Matrix/1
  p q r/1 -> Subsystem3/1(p q r1)
  Quaternions to Rotation Angles/1 -> Selector/1
  Selector/1 -> Euler/1
  Initial Euler Angles/1 -> Selector1/1
  Quaternions to Direction Cosine Matrix/1 -> DCM/1

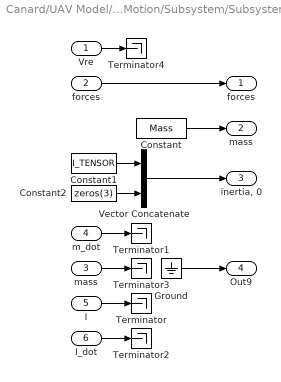
== system Canard/UAV Model/Equations of Motion/Subsystem/Subsystem2 ==
  Vre : Inport  OutDataTypeStr=double
  forces : Inport  Port=2  OutDataTypeStr=double
  "mass " : Inport  Port=3  OutDataTypeStr=double
  m_dot : Inport  Port=4  OutDataTypeStr=double
  I : Inport  Port=5  OutDataTypeStr=double
  I_dot : Inport  Port=6  OutDataTypeStr=double
  Constant : Constant  Value=Mass  OutDataTypeStr=Inherit: Inherit via back propagation
  Constant1 : Constant  Value=I_TENSOR  OutDataTypeStr=Inherit: Inherit via back propagation
  Constant2 : Constant  Value=zeros(3)
  Ground : Ground
  Terminator{,1..4} (5 alike) : Terminator
  Vector Concatenate : Concatenate  Mode=Multidimensional array
  "forces " : Outport  OutDataTypeStr=double  VectorParamsAs1DForOutWhenUnconnected=off
  mass : Outport  Port=2  OutDataTypeStr=double  VectorParamsAs1DForOutWhenUnconnected=off
  "inertia, 0" : Outport  Port=3  OutDataTypeStr=double  VectorParamsAs1DForOutWhenUnconnected=off
  Out9 : Outport  Port=4  OutDataTypeStr=double  VectorParamsAs1DForOutWhenUnconnected=off
  wires:
  m_dot/1 -> Terminator1/1
  forces/1 -> "forces "/1
  Constant/1 -> mass/1
  I_dot/1 -> Terminator2/1
  "mass "/1 -> Terminator3/1
  Constant2/1 -> Vector Concatenate/2
  Vre/1 -> Terminator4/1
  Ground/1 -> Out9/1
  I/1 -> Terminator/1
  Vector Concatenate/1 -> "inertia, 0"/1
  Constant1/1 -> Vector Concatenate/1

== system Canard/UAV Model/Equations of Motion/parameter/Acceleration ==
  note: 注意：
      | （1）三轴加速度并不等于速度的导数，这里的三轴加速度是传感器感受到的，包括飞机的机动
      | （2）过载定义为飞行员收到的除了重力以外的合力
  Ab : Inport
  Demux1 : Demux  Outputs=3
  Unary Minus1 : UnaryMinus
  ax : Outport
  ay : Outport  Port=2
  az : Outport  Port=3
  wires:
  Ab/1 -> Demux1/1
  Demux1/1 -> ax/1
  Demux1/2 -> ay/1
  Demux1/3 -> Unary Minus1/1
  Unary Minus1/1 -> az/1

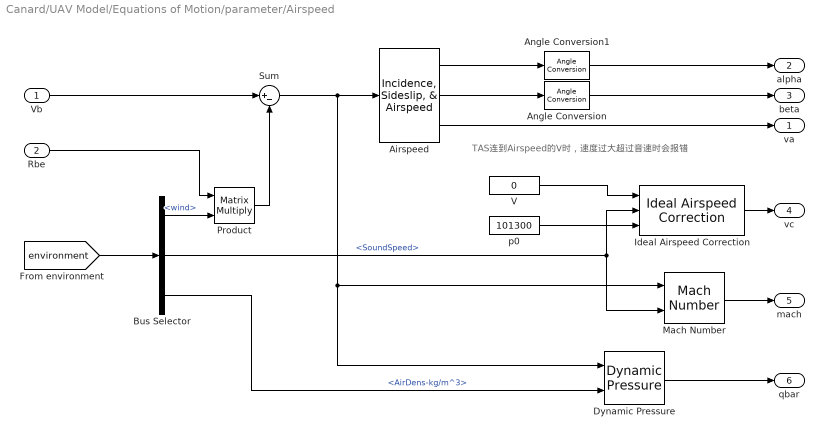
== system Canard/UAV Model/Equations of Motion/parameter/Airspeed ==
  note: TAS连到Airspeed的V时，速度过大超过音速时会报错
  Vb : Inport
  Rbe : Inport  Port=2
  Airspeed : aerolibasang/Incidence, Sideslip, & Airspeed
  Angle Conversion : aerolibconvert2/Angle Conversion  IU=rad  OU=deg
  Angle Conversion1 : aerolibconvert2/Angle Conversion  IU=rad  OU=deg
  Bus Selector : BusSelector  OutputSignals=wind,atmo.SoundSpeed,atmo.AirDens-kg/m^3
  Dynamic Pressure : aerolibasang/Dynamic Pressure
  Ideal Airspeed Correction : aerolibasang/Ideal Airspeed Correction  units=Metric (MKS)  vel_in=TAS  vel_out_tas=EAS  vel_out_eas=CAS  vel_out_cas=TAS  method=Table Lookup  SubOnly=off  action=Error
  Mach Number : aerolibasang/Mach Number
  Product : Product  Multiplication=Matrix(*)  RndMeth=Zero
  Sum : Sum  Inputs=|+-
  V : Constant  Value=0
  p0 : Constant  Value=101300
  va : Outport
  alpha : Outport  Port=2
  beta : Outport  Port=3
  vc : Outport  Port=4
  mach : Outport  Port=5
  qbar : Outport  Port=6
  wires:
  Mach Number/1 -> mach/1
  Dynamic Pressure/1 -> qbar/1
  Vb/1 -> Sum/1
  Rbe/1 -> Product/1
  Product/1 -> Sum/2
  Bus Selector/3 -> Dynamic Pressure/2  "<AirDens-kg/m^3>"
  Airspeed/3 -> va/1
  Ideal Airspeed Correction/1 -> vc/1
  Airspeed/1 -> Angle Conversion1/1
  Airspeed/2 -> Angle Conversion/1
  p0/1 -> Ideal Airspeed Correction/3
  Angle Conversion/1 -> beta/1
  Angle Conversion1/1 -> alpha/1
  [environment] -> Bus Selector/1
  Bus Selector/1 -> Product/2  "<wind>"
  Sum/1 -> Dynamic Pressure/1, Mach Number/1, Airspeed/1
  V/1 -> Ideal Airspeed Correction/1
  Bus Selector/2 -> Mach Number/2, Ideal Airspeed Correction/2  "<SoundSpeed>"

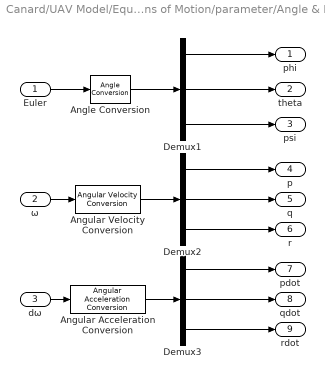
== system Canard/UAV Model/Equations of Motion/parameter/Angle & Rate ==
  Euler : Inport
  ω : Inport  Port=2
  dω : Inport  Port=3
  Angle Conversion : aerolibconvert2/Angle Conversion  IU=rad  OU=deg
  Angular Acceleration Conversion : aerolibconvert2/Angular Acceleration Conversion  IU=rad/s^2  OU=deg/s^2
  Angular Velocity Conversion : aerolibconvert2/Angular Velocity Conversion  IU=rad/s  OU=deg/s
  Demux1 : Demux  Outputs=3
  Demux2 : Demux  Outputs=3
  Demux3 : Demux  Outputs=3
  phi : Outport
  theta : Outport  Port=2
  psi : Outport  Port=3
  p : Outport  Port=4
  q : Outport  Port=5
  r : Outport  Port=6
  pdot : Outport  Port=7
  qdot : Outport  Port=8
  rdot : Outport  Port=9
  wires:
  Euler/1 -> Angle Conversion/1
  ω/1 -> Angular Velocity Conversion/1
  dω/1 -> Angular Acceleration Conversion/1
  Demux1/1 -> phi/1
  Demux1/2 -> theta/1
  Demux1/3 -> psi/1
  Demux2/1 -> p/1
  Demux2/2 -> q/1
  Demux2/3 -> r/1
  Demux3/1 -> pdot/1
  Demux3/2 -> qdot/1
  Demux3/3 -> rdot/1
  Angle Conversion/1 -> Demux1/1
  Angular Velocity Conversion/1 -> Demux2/1
  Angular Acceleration Conversion/1 -> Demux3/1

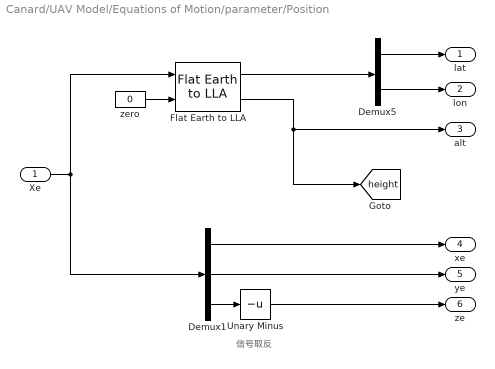
== system Canard/UAV Model/Equations of Motion/parameter/Position  ==
  note: 信号取反
  Xe : Inport
  Demux1 : Demux  Outputs=3
  Demux5 : Demux  Outputs=2
  Flat Earth to LLA : aerolibtransform2/Flat Earth to LLA  units=Metric (MKS)  ptype=Earth (WGS84)  F=1/298.257223563  R=6378137  refPosPort=off  LL0=[0 10]  psi=0
  Unary Minus : UnaryMinus
  zero : Constant  Value=0
  lat : Outport
  lon : Outport  Port=2
  alt : Outport  Port=3
  xe : Outport  Port=4
  ye : Outport  Port=5
  ze : Outport  Port=6
  tag scope: height=global
  wires:
  Flat Earth to LLA/2 -> alt/1, [height]
  zero/1 -> Flat Earth to LLA/2
  Flat Earth to LLA/1 -> Demux5/1
  Demux5/1 -> lat/1
  Demux5/2 -> lon/1
  Demux1/1 -> xe/1
  Demux1/2 -> ye/1
  Demux1/3 -> Unary Minus/1
  Xe/1 -> Demux1/1, Flat Earth to LLA/1
  Unary Minus/1 -> ze/1

== system Canard/UAV Model/Equations of Motion/parameter/Speed ==
  Ve : Inport
  Demux2 : Demux  Outputs=3
  Unary Minus : UnaryMinus
  vx : Outport
  vy : Outport  Port=2
  vz : Outport  Port=3
  wires:
  Ve/1 -> Demux2/1
  Demux2/1 -> vx/1
  Demux2/2 -> vy/1
  Demux2/3 -> Unary Minus/1
  Unary Minus/1 -> vz/1

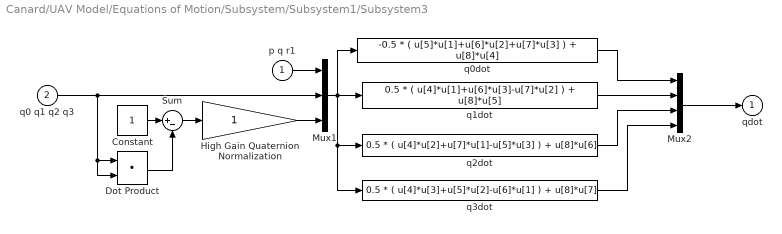
== system Canard/UAV Model/Equations of Motion/Subsystem/Subsystem1/Subsystem3 ==
  p q r1 : Inport
  q0 q1 q2 q3 : Inport  Port=2
  Constant : Constant
  Dot Product : DotProduct  InputSameDT=off  OutDataTypeStr=Inherit: Inherit via internal rule
  High Gain Quaternion Normalization : Gain  SaturateOnIntegerOverflow=on  OutDataTypeStr=Inherit: Same as input  ParamDataTypeStr=Inherit: Same as input
  Mux1 : Mux  Inputs=[3 4 1]
  Mux2 : Mux
  Sum : Sum  Inputs=|+-  InputSameDT=on  SaturateOnIntegerOverflow=on  OutDataTypeStr=Inherit: Same as first input
  q0dot : Fcn  Expr=-0.5 * ( u[5]*u[1]+u[6]*u[2]+u[7]*u[3] ) + u[8]*u[4]
  q1dot : Fcn  Expr=0.5 * ( u[4]*u[1]+u[6]*u[3]-u[7]*u[2] ) + u[8]*u[5]
  q2dot : Fcn  Expr=0.5 * ( u[4]*u[2]+u[7]*u[1]-u[5]*u[3] ) + u[8]*u[6]
  q3dot : Fcn  Expr=0.5 * ( u[4]*u[3]+u[5]*u[2]-u[6]*u[1] ) + u[8]*u[7]
  qdot : Outport  InitialOutput=0  VectorParamsAs1DForOutWhenUnconnected=off
  wires:
  Mux1/1 -> q2dot/1, q3dot/1, q0dot/1, q1dot/1
  q1dot/1 -> Mux2/2
  q0 q1 q2 q3/1 -> Dot Product/1, Dot Product/2, Mux1/2
  Dot Product/1 -> Sum/2
  Sum/1 -> High Gain Quaternion Normalization/1
  p q r1/1 -> Mux1/1
  Mux2/1 -> qdot/1
  High Gain Quaternion Normalization/1 -> Mux1/3
  q3dot/1 -> Mux2/4
  Constant/1 -> Sum/1
  q0dot/1 -> Mux2/1
  q2dot/1 -> Mux2/3

== matlab function Canard/NDI Control Law/MATLAB Function ==
  data: u input; De output
function De = M2De(u)
%#codegen

M=u(1);%N*m
V=u(2);%m/s
alpha=u(3);%deg
qbar=u(4);%pa
q=u(5);%deg/s

S=1.485;
cbar=0.552;

cm0 = -0.0037; cm_q = -0.082; cm_de = -0.0155;
De=(M*(inv(qbar*S*cbar))-cm0-(cbar/(2*V))*cm_q*q)*(inv(cm_de));

== matlab function Canard/NDI Control Law/MATLAB Function1 ==
  data: thetac_dot input; q_c output; phi input; r input
function q_c = fcn(thetac_dot,phi,r)
%#codegen

q_c=(inv(cosd(phi)))*(thetac_dot+r*sind(phi));

== matlab function Canard/NDI Control Law/MATLAB Function2 ==
  data: Vdot input; DT output; Gx input
function DT = fcn(Vdot,Gx)
max_T = 97.02;
m=18;
DT=(m*Vdot-Gx)/max_T;

== matlab function Canard/NDI Control Law/Subsystem/MATLAB Function ==
  data: p input; r input; q_dot input; M output
function M = fcn(p,r,q_dot)
%#codegen
I_x=2.9;
I_y=3.1;
I_z=2.5;
I_xz=0;
c5=(I_z-I_x)/I_y;
c6=I_xz/I_y;
c7=1/I_y;

M=(inv(c7))*(q_dot-c5*p*r+c6*(p*p-r*r));

== matlab function Canard/NDI Control Law/Subsystem1/MATLAB Function ==
  data: p input; L output; q input; r input; p_dot input; r_dot input; N output
function [L,N] = fcn(p,q,r,p_dot,r_dot)
I_x=2.9;
I_y=3.1;
I_z=2.5;
I_xz=0;

c1=((I_y-I_z)*I_z-I_xz^2)/(I_x*I_z-I_xz^2);
c2=((I_x-I_y+I_z)*I_xz)/(I_x*I_z-I_xz^2);
c3=I_z/(I_x*I_z-I_xz^2);
c4=I_xz/(I_x*I_z-I_xz^2);
c8=(I_x*(I_x-I_y)+I_xz^2)/(I_x*I_z-I_xz^2);
c9=I_x/(I_x*I_z-I_xz^2);

g1_lat=[c3 c4;c4 c9];
f1_lat=[(c1*r+c2*p)*q;(c8*p-c2*r)*q];
v1_lat=[p_dot;r_dot];

LN=(inv(g1_lat))*(v1_lat-f1_lat);
L=LN(1,:);
N=LN(2,:);

%#codegen

== matlab function Canard/NDI Control Law/Subsystem2/MATLAB Function ==
  data: qbar input; Da output; alpha input; beta input; va input; p input; r input; L input; N input; Dr output
function [Da,Dr] = fcn(qbar,alpha,beta,va,p,r,L,N)
%#codegen
S=1.485;%m^2
bar=3.0;%m

croll=L/(qbar*S*bar);
cn=N/(qbar*S*bar);

croll_b = -0.0016; croll_p = -0.0071; croll_r = 0.0023; croll_da = -0.0012; croll_dr = 2.2387e-4;
cn_b = 0.0017; cn_p = -0.0011; cn_r = -0.0031; cn_da = 3.8171e-5; cn_dr = -0.0012;
f=[croll_b*beta+(bar/(2*va))*croll_p*p+(bar/(2*va))*croll_r*r;...
    cn_b*beta+(bar/(2*va))*cn_p*p+(bar/(2*va))*cn_r*r];
g=[croll_da croll_dr;cn_da cn_dr];
croll_cn=[croll;cn];

DaDr=(inv(g))*(croll_cn-f);
Da=DaDr(1,:);
Dr=DaDr(2,:);

== matlab function Canard/NDI Control Law/Subsystem3/MATLAB Function ==
  data: phi_dot input; p_c output; psi_dot input; theta input; phi input; q input; r_c output
function [p_c,r_c] = fcn(phi_dot,psi_dot,theta,phi,q)
%#codegen

f=[q*tand(theta)*sind(phi);q*sind(phi)/cosd(theta)];
g=[1,tand(theta)*cosd(phi);0,cosd(phi)/cosd(theta)];
v=[phi_dot;psi_dot];

pr=(inv(g))*(v-f);

p_c=pr(1,:);
r_c=pr(2,:);

== matlab function Canard/UAV Model/gravitation/MATLAB Function ==
  data: u input; Gx output; Gy output; Gz output
function [Gx,Gy,Gz]= fcn(u)
%#codegen
G=u(1);
theta=u(2);
phi=u(3);
Gx=-G*sind(theta);
Gy=G*cosd(theta)*sind(phi);
Gz=G*cosd(theta)*cosd(phi);
